simulink model "nms_3Dmodel"  (R2017b)
settings: Solver=ode15s  StartTime=0.0  StopTime=t_end  FixedStep=1e-3  RelTol=1e-3  AbsTol=1e-4  EnableMultiTasking=on
InitFcn:
  | runScripts;
values from neighbouring files (symbols this model uses):
  ankle_height = 0.08    [nms_MechInit.m]
  ankleIMP = param(91+length(paramIC_opt):93+length(paramIC_opt))    [runScripts.m]
  c = 0.05    [IID_nms_MechInit.m]    (also in nms_MechInit.m)
  c_jointstop = 0.3 / (pi/180)    (= 17.1887338539)    [IID_nms_MechInit.m]    (also in nms_MechInit.m)
  CtrlPar_FP = [alpha0 alpha_cd alpha_cv]    [setCtrlPar.m]
  CtrlPar_FP_R = [R_hipR0 R_hipR_cd R_hipR_cv]    [setCtrlPar.m]
  CtrlPar_LL = l_clr    [setCtrlPar.m]
  CtrlPar_St = [StPreStim St_M1 St_M2 St_M3 St_M4 St_M5 St_M11]    [setCtrlPar.m]
  CtrlPar_St_R = [R_StPreStim R_St_M1 R_St_M3 R_St_M4]    [setCtrlPar.m]
  CtrlPar_Sw = [SwPreStim SwPhasePari SwPhaseParii SwCtrlPar_H SwCtrlPar_A      SwCtrlPar_Ki SwCtrlPar_Kii SwCtrlPar_Kiii SwCtrlPar_StP]    [setCtrlPar.m]
  CtrlPar_Sw_R = [R_SwPreStim R_Sw_M6]    [setCtrlPar.m]
  CtrlPar_theta0 = parBlCtrl(1)      *1*pi/180    [setCtrlPar.m]
  CtrlPar_Tr = [Tr_St_sup Tr_Sw]    [setCtrlPar.m]
  CtrlPar_Tr_R = [R_Tr_St_sup R_Tr_Sw]    [setCtrlPar.m]
  D12_F = 0.16    [IID_nms_MechInit.m]    (also in nms_MechInit.m)
  D12_S = L_S    (= 0.5)    [IID_nms_MechInit.m]    (also in nms_MechInit.m = 0.46)
  D12_T = L_T    (= 0.5)    [IID_nms_MechInit.m]    (also in nms_MechInit.m = 0.46)
  D12z_T = 0.1* scalorFactor    (= 0.1)    [nms_MechInit.m]
  D13_F = 0.20    (= 0.2)    [IID_nms_MechInit.m]    (also in nms_MechInit.m)
  D1G_F = 0.14    [IID_nms_MechInit.m]    (also in nms_MechInit.m)
  D1G_HAT = 0.35    [IID_nms_MechInit.m]    (also in nms_MechInit.m)
  D1G_S = 0.3    [IID_nms_MechInit.m]    (also in nms_MechInit.m = 0.28)
  D1G_T = 0.3    [IID_nms_MechInit.m]    (also in nms_MechInit.m = 0.28)
  D1Gy_F = ankle_height*D1G_F/D12_F    (= 0.07)    [nms_MechInit.m]
  d_fBall = 0.1    [nms_MechInit.m]
  d_fHeel = 0.05    [nms_MechInit.m]
  DeltaThRef = 5e-3    (= 0.005)    [IID_nms_MechInit.m]    (also in nms_MechInit.m)
  Dist_LM23_PH = 0    [setDistPar.m]
  Dist_LM34_PH = 0    [setDistPar.m]
  Dist_On = 1    [IID_setDistPar.m]    (also in setDistPar.m)
  Dist_PDur = 0.15    [IID_setDistPar.m]    (also in setDistPar.m)
  Dist_RM23_PH = 0    [setDistPar.m]
  Dist_RM34_PH = 0    [setDistPar.m]
  Dist_StartTime = 15    [IID_setDistPar.m]    (also in setDistPar.m)
  Dist_xyzHAT_front_PH = 0    [setDistPar.m]
  Dist_xyzHAT_sag_PH = 0    [IID_setDistPar.m]    (also in setDistPar.m)
  Dist_xyzLAnkle_PH = 0    [setDistPar.m]
  Dist_xyzRAnkle_PH = 0    [setDistPar.m]
  eref = 0.04    [IID_nms_MechInit.m]    (also in nms_MechInit.m)
  FmaxBFSH = 350    [nms_MechInit.m]
  FmaxGAS = 1500    [IID_nms_MechInit.m]    (also in nms_MechInit.m)
  FmaxGLU = 1500    [IID_nms_MechInit.m]    (also in nms_MechInit.m)
  FmaxHAB = 3000    [nms_MechInit.m]
  FmaxHAD = 4500    [nms_MechInit.m]
  FmaxHAM = 3000    [IID_nms_MechInit.m]    (also in nms_MechInit.m)
  FmaxHFL = 2000    [IID_nms_MechInit.m]    (also in nms_MechInit.m)
  FmaxRF = 1200    [nms_MechInit.m]
  FmaxSOL = 4000    [IID_nms_MechInit.m]    (also in nms_MechInit.m)
  FmaxTA = 800    [IID_nms_MechInit.m]    (also in nms_MechInit.m)
  FmaxVAS = 6000    [IID_nms_MechInit.m]    (also in nms_MechInit.m)
  In_F = 0.005    [IID_nms_MechInit.m]    (also in nms_MechInit.m)
  In_HAT = 3    [IID_nms_MechInit.m]    (also in nms_MechInit.m = 2.5)
  In_S = 0.05    [IID_nms_MechInit.m]    (also in nms_MechInit.m)
  In_T = 0.15    [IID_nms_MechInit.m]    (also in nms_MechInit.m)
  init_a_tgt = 70*pi/180    (= 1.2217304764)    [setInitPar.m]
  init_a_tgtR = 90*pi/180    (= 1.57079632679)    [setInitPar.m]
  Inx_F = 0.0007    [nms_MechInit.m]
  Inx_HAT = 1.0    (= 1)    [nms_MechInit.m]
  Inx_S = 0.003    [nms_MechInit.m]
  Inx_T = 0.03    [nms_MechInit.m]
  Iny_F = 0.005    [nms_MechInit.m]
  Iny_HAT = 4.0    (= 4)    [nms_MechInit.m]
  Iny_S = 0.05    [nms_MechInit.m]
  Iny_T = 0.15    [nms_MechInit.m]
  K = 5    [IID_nms_MechInit.m]    (also in nms_MechInit.m)
  k_gn = k_gn/2    (= 39240)    [nms_MechInit.m]
  k_gt = k_gt/2    (= 3924)    [nms_MechInit.m]
  k_pressure = m_HAT * 9.81 / DeltaThRef    (= 104967)    [IID_nms_MechInit.m]    (also in nms_MechInit.m)
  leg_l = [D12_T D12_S]    [nms_MechInit.m]
  LongDelay = 0.020    (= 0.02)    [IID_setCtrlPar.m]    (also in nms_MechInit.m = 0.01)
  LongLoopDelay = 0.030    (= 0.03)    [nms_MechInit.m]
  loptBFSH = 0.12    [nms_MechInit.m]
  loptGAS = 0.05    [IID_nms_MechInit.m]    (also in nms_MechInit.m)
  loptGLU = 0.11    [IID_nms_MechInit.m]    (also in nms_MechInit.m)
  loptHAB = 0.09    [nms_MechInit.m]
  loptHAD = 0.10    (= 0.1)    [nms_MechInit.m]
  loptHAM = 0.10    (= 0.1)    [IID_nms_MechInit.m]    (also in nms_MechInit.m)
  loptHFL = 0.11    [IID_nms_MechInit.m]    (also in nms_MechInit.m)
  loptRF = 0.08    [nms_MechInit.m]
  loptSOL = 0.04    [IID_nms_MechInit.m]    (also in nms_MechInit.m)
  loptTA = 0.06    [IID_nms_MechInit.m]    (also in nms_MechInit.m)
  loptVAS = 0.08    [IID_nms_MechInit.m]    (also in nms_MechInit.m)
  lslackBFSH = 0.10    (= 0.1)    [nms_MechInit.m]
  lslackGAS = 0.40    (= 0.4)    [IID_nms_MechInit.m]    (also in nms_MechInit.m)
  lslackGLU = 0.13    [IID_nms_MechInit.m]    (also in nms_MechInit.m)
  lslackHAB = 0.07    [nms_MechInit.m]
  lslackHAD = 0.18    [nms_MechInit.m]
  lslackHAM = 0.31    [IID_nms_MechInit.m]    (also in nms_MechInit.m)
  lslackHFL = 0.10    (= 0.1)    [IID_nms_MechInit.m]    (also in nms_MechInit.m)
  lslackRF = 0.35    [nms_MechInit.m]
  lslackSOL = 0.26    [IID_nms_MechInit.m]    (also in nms_MechInit.m)
  lslackTA = 0.24    [IID_nms_MechInit.m]    (also in nms_MechInit.m)
  lslackVAS = 0.23    [IID_nms_MechInit.m]    (also in nms_MechInit.m)
  m_F = 1.25    [IID_nms_MechInit.m]    (also in nms_MechInit.m)
  m_HAT = 53.5    [IID_nms_MechInit.m]    (also in nms_MechInit.m)
  m_S = 3.5    [IID_nms_MechInit.m]    (also in nms_MechInit.m)
  m_T = 8.5    [IID_nms_MechInit.m]    (also in nms_MechInit.m)
  m_Total = m_F*2+m_S*2+m_T*2+m_HAT    (= 80)    [IID_nms_MechInit.m]    (also in nms_MechInit.m)
  massBFSH = 2    [nms_MechInit.m]
  massGAS = 0.45    [IID_nms_MechInit.m]    (also in nms_MechInit.m)
  massGLU = 1.4    [IID_nms_MechInit.m]    (also in nms_MechInit.m)
  massHAB = 1.145    [nms_MechInit.m]
  massHAD = 1.91    [nms_MechInit.m]
  massHAM = 1.82    [IID_nms_MechInit.m]    (also in nms_MechInit.m)
  massHFL = 1.87    [IID_nms_MechInit.m]    (also in nms_MechInit.m)
  massRF = 1    [nms_MechInit.m]
  massSOL = 1.36    [IID_nms_MechInit.m]    (also in nms_MechInit.m)
  massTA = 0.29    [IID_nms_MechInit.m]    (also in nms_MechInit.m)
  massVAS = 2.91    [IID_nms_MechInit.m]    (also in nms_MechInit.m)
  MidDelay = 0.010    (= 0.01)    [IID_setCtrlPar.m]    (also in nms_MechInit.m = 0.005)
  mu_slide = 0.8    [IID_nms_MechInit.m]    (also in nms_MechInit.m)
  mu_stick = 0.9    [IID_nms_MechInit.m]    (also in nms_MechInit.m)
  N = 1.5    [IID_nms_MechInit.m]    (also in cmaes_parfor.m = size(x,1); nms_MechInit.m)
  Passive_ankle = 1    [runScripts.m]
  phi12_LowLimit = 70*pi/180    (= 1.2217304764)    [IID_nms_MechInit.m]    (also in nms_MechInit.m)
  phi12_UpLimit = 130*pi/180    (= 2.26892802759)    [IID_nms_MechInit.m]    (also in nms_MechInit.m)
  phi23_UpLimit = 175*pi/180    (= 3.05432619099)    [IID_nms_MechInit.m]    (also in nms_MechInit.m)
  phi34_UpLimit = 230*pi/180    (= 4.01425727959)    [IID_nms_MechInit.m]    (also in nms_MechInit.m)
  phi34R_LowLimit = -15*pi/180    (= -0.261799387799)    [nms_MechInit.m]
  phi34R_UpLimit = 50*pi/180    (= 0.872664625997)    [nms_MechInit.m]
  ... (+114 more)
undefined symbols (not defined in the file or in its folder): magnitude, sgn
libraries: mblibv1 x104, simulink x50, simulink_extras x38, nmc x30
(part 5 of 16)

== system nms_3Dmodel/Body Mechanics Layer/LLHeelCnt5 ==
  note: 3D Ground Interaction Model
  PosContra : Inport
  3D Contact : Subsystem
  Body Actuator : mblibv1/Sensors &  Actuators/Body Actuator  UpdateFromCAD=off  PhysicalDomain=Mechanical  PortType=blob  ActuationStyle=Force  AngleUnits=deg  ArcVelocityUnits=deg/s  ArcAccelerationUnits=deg/s^2  CoordPositionUnits=m  VelocityUnits=m/s  AccelerationUnits=m/s^2  ForceUnits=N  TorqueUnits=N*m  ActiveIO=on  Width=3  DialogClass=MechanicalActuatorBlock  ReferenceFrame=Absolute (World)  Angle=off  CoordPosition=on  Force=on  Torque=off
      settings: SourceProductName=Simscape Multibody  SourceProductBaseCode=MS
  Body Sensor : mblibv1/Sensors &  Actuators/Body Sensor  UpdateFromCAD=off  PhysicalDomain=Mechanical  PortType=blob  Muxed=off  Pose=off  Angle=on  AngleUnits=deg  ArcVelocity=off  ArcVelocityUnits=deg/s  ArcAcceleration=off  ArcAccelerationUnits=deg/s^2  CoordPosition=on  CoordPositionUnits=m  Velocity=on  VelocityUnits=m/s  Acceleration=off  AccelerationUnits=m/s^2  Quaternion=on  QuaternionDT=off  QuaternionDDT=off  QuaternionUnits=off  OutputVector=[ 3 3 ]  ActiveIO=on  Width=6  DialogClass=MechanicalSensorBlock  ReferenceFrame=Absolute (World)
      settings: SourceProductName=Simscape Multibody  SourceProductBaseCode=MS
  Demux1 : Demux  Outputs=3
  GroundFunction : nmc/GroundFunction
      settings: SourceProductName=Neuro Muscular Controller Library
  Mechanical Branching Bar : mblibv1/Utilities/Mechanical Branching Bar  LConnTagsString=_newl0  RConnTagsString=SA0|SA1  UpdateFromCAD=off  DialogClass=MechanicalBranchingBarBlock  NumSAPorts=2
      settings: SourceProductName=Simscape Multibody  SourceProductBaseCode=MS
  Mux : Mux  Inputs=3
  Sum : Sum  Inputs=|+-
  Sum1 : Sum
  Terminator : Terminator
  contact? : simulink/Logic and Bit Operations/Compare To Zero  relop=<=  OutDataTypeStr=boolean
  y : Selector  InputPortWidth=3  IndexOptions=Index vector (dialog)  Indices=2  OutputSizes=1
  F : PMIOPort  Port=1  Side=Left
  RBallCnt : Outport
  tag scope: GRF_LLHeelCnt5=global
  wires:
  GroundFunction/2 -> 3D Contact/2(nVec [m m m])
  GroundFunction/1 -> Mux/2, Sum/2
  Demux1/2 -> Terminator/1
  Demux1/3 -> Mux/3
  Demux1/1 -> Mux/1
  Mux/1 -> 3D Contact/1(RefPt [m m m])  "Reference Point RefPt"
  y/1 -> Sum/1
  Sum/1 -> contact?/1
  3D Contact/2(FtVec [N N N]) -> Sum1/2
  3D Contact/1(FnVec [N N N]) -> Sum1/1
  Body Sensor/2 -> 3D Contact/4(vVec [m/s m/s m/s])
  Body Sensor/1 -> y/1, Demux1/1, 3D Contact/3(pVec [m m m])  "pos"
  contact?/1 -> RBallCnt/1, 3D Contact/Enable  "cnt"
  PosContra/1 -> GroundFunction/1
  Sum1/1 -> [GRF_LLHeelCnt5], Body Actuator/1
  connections:
  Mechanical Branching Bar/RConn1 -- Body Sensor/LConn1
  Mechanical Branching Bar/RConn2 -- Body Actuator/RConn1
  F/RConn1 -- Mechanical Branching Bar/LConn1

== system nms_3Dmodel/Body Mechanics Layer/LLHeelCnt6 ==
  note: 3D Ground Interaction Model
  PosContra : Inport
  3D Contact : Subsystem
  Body Actuator : mblibv1/Sensors &  Actuators/Body Actuator  UpdateFromCAD=off  PhysicalDomain=Mechanical  PortType=blob  ActuationStyle=Force  AngleUnits=deg  ArcVelocityUnits=deg/s  ArcAccelerationUnits=deg/s^2  CoordPositionUnits=m  VelocityUnits=m/s  AccelerationUnits=m/s^2  ForceUnits=N  TorqueUnits=N*m  ActiveIO=on  Width=3  DialogClass=MechanicalActuatorBlock  ReferenceFrame=Absolute (World)  Angle=off  CoordPosition=on  Force=on  Torque=off
      settings: SourceProductName=Simscape Multibody  SourceProductBaseCode=MS
  Body Sensor : mblibv1/Sensors &  Actuators/Body Sensor  UpdateFromCAD=off  PhysicalDomain=Mechanical  PortType=blob  Muxed=off  Pose=off  Angle=on  AngleUnits=deg  ArcVelocity=off  ArcVelocityUnits=deg/s  ArcAcceleration=off  ArcAccelerationUnits=deg/s^2  CoordPosition=on  CoordPositionUnits=m  Velocity=on  VelocityUnits=m/s  Acceleration=off  AccelerationUnits=m/s^2  Quaternion=on  QuaternionDT=off  QuaternionDDT=off  QuaternionUnits=off  OutputVector=[ 3 3 ]  ActiveIO=on  Width=6  DialogClass=MechanicalSensorBlock  ReferenceFrame=Absolute (World)
      settings: SourceProductName=Simscape Multibody  SourceProductBaseCode=MS
  Demux1 : Demux  Outputs=3
  GroundFunction : nmc/GroundFunction
      settings: SourceProductName=Neuro Muscular Controller Library
  Mechanical Branching Bar : mblibv1/Utilities/Mechanical Branching Bar  LConnTagsString=_newl0  RConnTagsString=SA0|SA1  UpdateFromCAD=off  DialogClass=MechanicalBranchingBarBlock  NumSAPorts=2
      settings: SourceProductName=Simscape Multibody  SourceProductBaseCode=MS
  Mux : Mux  Inputs=3
  Sum : Sum  Inputs=|+-
  Sum1 : Sum
  Terminator : Terminator
  contact? : simulink/Logic and Bit Operations/Compare To Zero  relop=<=  OutDataTypeStr=boolean
  y : Selector  InputPortWidth=3  IndexOptions=Index vector (dialog)  Indices=2  OutputSizes=1
  F : PMIOPort  Port=1  Side=Left
  RBallCnt : Outport
  tag scope: GRF_LLHeelCnt6=global
  wires:
  GroundFunction/2 -> 3D Contact/2(nVec [m m m])
  GroundFunction/1 -> Mux/2, Sum/2
  Demux1/2 -> Terminator/1
  Demux1/3 -> Mux/3
  Demux1/1 -> Mux/1
  Mux/1 -> 3D Contact/1(RefPt [m m m])  "Reference Point RefPt"
  y/1 -> Sum/1
  Sum/1 -> contact?/1
  3D Contact/2(FtVec [N N N]) -> Sum1/2
  3D Contact/1(FnVec [N N N]) -> Sum1/1
  Body Sensor/2 -> 3D Contact/4(vVec [m/s m/s m/s])
  Body Sensor/1 -> y/1, Demux1/1, 3D Contact/3(pVec [m m m])  "pos"
  contact?/1 -> RBallCnt/1, 3D Contact/Enable  "cnt"
  PosContra/1 -> GroundFunction/1
  Sum1/1 -> [GRF_LLHeelCnt6], Body Actuator/1
  connections:
  Mechanical Branching Bar/RConn1 -- Body Sensor/LConn1
  Mechanical Branching Bar/RConn2 -- Body Actuator/RConn1
  F/RConn1 -- Mechanical Branching Bar/LConn1

== system nms_3Dmodel/Body Mechanics Layer/LLHeelCnt7 ==
  note: 3D Ground Interaction Model
  3D Contact : Subsystem
  Body Actuator : mblibv1/Sensors &  Actuators/Body Actuator  UpdateFromCAD=off  PhysicalDomain=Mechanical  PortType=blob  ActuationStyle=Force  AngleUnits=deg  ArcVelocityUnits=deg/s  ArcAccelerationUnits=deg/s^2  CoordPositionUnits=m  VelocityUnits=m/s  AccelerationUnits=m/s^2  ForceUnits=N  TorqueUnits=N*m  ActiveIO=on  Width=3  DialogClass=MechanicalActuatorBlock  ReferenceFrame=Absolute (World)  Angle=off  CoordPosition=on  Force=on  Torque=off
      settings: SourceProductName=Simscape Multibody  SourceProductBaseCode=MS
  Body Sensor : mblibv1/Sensors &  Actuators/Body Sensor  UpdateFromCAD=off  PhysicalDomain=Mechanical  PortType=blob  Muxed=off  Pose=off  Angle=on  AngleUnits=deg  ArcVelocity=off  ArcVelocityUnits=deg/s  ArcAcceleration=off  ArcAccelerationUnits=deg/s^2  CoordPosition=on  CoordPositionUnits=m  Velocity=on  VelocityUnits=m/s  Acceleration=off  AccelerationUnits=m/s^2  Quaternion=on  QuaternionDT=off  QuaternionDDT=off  QuaternionUnits=off  OutputVector=[ 3 3 ]  ActiveIO=on  Width=6  DialogClass=MechanicalSensorBlock  ReferenceFrame=Absolute (World)
      settings: SourceProductName=Simscape Multibody  SourceProductBaseCode=MS
  Demux1 : Demux  Outputs=3
  GroundFunction : nmc/GroundFunction
      settings: SourceProductName=Neuro Muscular Controller Library
  Mechanical Branching Bar : mblibv1/Utilities/Mechanical Branching Bar  LConnTagsString=_newl0  RConnTagsString=SA0|SA1  UpdateFromCAD=off  DialogClass=MechanicalBranchingBarBlock  NumSAPorts=2
      settings: SourceProductName=Simscape Multibody  SourceProductBaseCode=MS
  Mux : Mux  Inputs=3
  Sum : Sum  Inputs=|+-
  Sum1 : Sum
  Terminator : Terminator
  contact? : simulink/Logic and Bit Operations/Compare To Zero  relop=<=  OutDataTypeStr=boolean
  y : Selector  InputPortWidth=3  IndexOptions=Index vector (dialog)  Indices=2  OutputSizes=1
  F : PMIOPort  Port=1  Side=Left
  RBallCnt : Outport
  RBallCnt1 : Outport  Port=2
  tag scope: GRF_LLHeelCnt7=global
  wires:
  contact?/1 -> 3D Contact/Enable, RBallCnt/1  "cnt"
  Body Sensor/1 -> RBallCnt1/1, GroundFunction/1, 3D Contact/3(pVec [m m m]), Demux1/1, y/1  "pos"
  Body Sensor/2 -> 3D Contact/4(vVec [m/s m/s m/s])
  3D Contact/1(FnVec [N N N]) -> Sum1/1
  3D Contact/2(FtVec [N N N]) -> Sum1/2
  Sum/1 -> contact?/1
  y/1 -> Sum/1
  Mux/1 -> 3D Contact/1(RefPt [m m m])  "Reference Point RefPt"
  Demux1/1 -> Mux/1
  Demux1/3 -> Mux/3
  Demux1/2 -> Terminator/1
  GroundFunction/1 -> Sum/2, Mux/2
  GroundFunction/2 -> 3D Contact/2(nVec [m m m])
  Sum1/1 -> [GRF_LLHeelCnt7], Body Actuator/1
  connections:
  F/RConn1 -- Mechanical Branching Bar/LConn1
  Mechanical Branching Bar/RConn2 -- Body Actuator/RConn1
  Mechanical Branching Bar/RConn1 -- Body Sensor/LConn1

== system nms_3Dmodel/Body Mechanics Layer/LLHeelCnt8 ==
  note: 3D Ground Interaction Model
  3D Contact : Subsystem
  Body Actuator : mblibv1/Sensors &  Actuators/Body Actuator  UpdateFromCAD=off  PhysicalDomain=Mechanical  PortType=blob  ActuationStyle=Force  AngleUnits=deg  ArcVelocityUnits=deg/s  ArcAccelerationUnits=deg/s^2  CoordPositionUnits=m  VelocityUnits=m/s  AccelerationUnits=m/s^2  ForceUnits=N  TorqueUnits=N*m  ActiveIO=on  Width=3  DialogClass=MechanicalActuatorBlock  ReferenceFrame=Absolute (World)  Angle=off  CoordPosition=on  Force=on  Torque=off
      settings: SourceProductName=Simscape Multibody  SourceProductBaseCode=MS
  Body Sensor : mblibv1/Sensors &  Actuators/Body Sensor  UpdateFromCAD=off  PhysicalDomain=Mechanical  PortType=blob  Muxed=off  Pose=off  Angle=on  AngleUnits=deg  ArcVelocity=off  ArcVelocityUnits=deg/s  ArcAcceleration=off  ArcAccelerationUnits=deg/s^2  CoordPosition=on  CoordPositionUnits=m  Velocity=on  VelocityUnits=m/s  Acceleration=off  AccelerationUnits=m/s^2  Quaternion=on  QuaternionDT=off  QuaternionDDT=off  QuaternionUnits=off  OutputVector=[ 3 3 ]  ActiveIO=on  Width=6  DialogClass=MechanicalSensorBlock  ReferenceFrame=Absolute (World)
      settings: SourceProductName=Simscape Multibody  SourceProductBaseCode=MS
  Demux1 : Demux  Outputs=3
  GroundFunction : nmc/GroundFunction
      settings: SourceProductName=Neuro Muscular Controller Library
  Mechanical Branching Bar : mblibv1/Utilities/Mechanical Branching Bar  LConnTagsString=_newl0  RConnTagsString=SA0|SA1  UpdateFromCAD=off  DialogClass=MechanicalBranchingBarBlock  NumSAPorts=2
      settings: SourceProductName=Simscape Multibody  SourceProductBaseCode=MS
  Mux : Mux  Inputs=3
  Sum : Sum  Inputs=|+-
  Sum1 : Sum
  Terminator : Terminator
  contact? : simulink/Logic and Bit Operations/Compare To Zero  relop=<=  OutDataTypeStr=boolean
  y : Selector  InputPortWidth=3  IndexOptions=Index vector (dialog)  Indices=2  OutputSizes=1
  F : PMIOPort  Port=1  Side=Left
  RBallCnt : Outport
  RBallCnt1 : Outport  Port=2
  tag scope: GRF_LLHeelCnt8=global
  wires:
  contact?/1 -> 3D Contact/Enable, RBallCnt/1  "cnt"
  Body Sensor/1 -> RBallCnt1/1, GroundFunction/1, 3D Contact/3(pVec [m m m]), Demux1/1, y/1  "pos"
  Body Sensor/2 -> 3D Contact/4(vVec [m/s m/s m/s])
  3D Contact/1(FnVec [N N N]) -> Sum1/1
  3D Contact/2(FtVec [N N N]) -> Sum1/2
  Sum/1 -> contact?/1
  y/1 -> Sum/1
  Mux/1 -> 3D Contact/1(RefPt [m m m])  "Reference Point RefPt"
  Demux1/1 -> Mux/1
  Demux1/3 -> Mux/3
  Demux1/2 -> Terminator/1
  GroundFunction/1 -> Sum/2, Mux/2
  GroundFunction/2 -> 3D Contact/2(nVec [m m m])
  Sum1/1 -> [GRF_LLHeelCnt8], Body Actuator/1
  connections:
  F/RConn1 -- Mechanical Branching Bar/LConn1
  Mechanical Branching Bar/RConn2 -- Body Actuator/RConn1
  Mechanical Branching Bar/RConn1 -- Body Sensor/LConn1

== system nms_3Dmodel/Body Mechanics Layer/Left Leg Load ==
  dxThigh [m] : Inport
  FB Gain1 : Gain  Gain=1/DeltaThRef  SaturateOnIntegerOverflow=on  OutDataTypeStr=Inherit: Same as input  ParamDataTypeStr=Inherit: Same as input
  Saturation11 : Saturate  UpperLimit=inf  LowerLimit=0  ZeroCross=off
  smooth2 : TransferFcn  Denominator=[0.02 1]
  LLoad [F] : Outport
  wires:
  Saturation11/1 -> FB Gain1/1
  smooth2/1 -> Saturation11/1
  FB Gain1/1 -> LLoad [F]/1
  dxThigh [m]/1 -> smooth2/1

== system nms_3Dmodel/Body Mechanics Layer/Left Thigh Sensor Sheet ==
  note: Inner Segment Pressure Sheet
  Gain3 : Gain  Gain=k_pressure
  Gain4 : Gain  Gain=1/v_max_pressure
  Inner Thigh Shift Joint : mblibv1/Joints/Prismatic  LConnTagsString=__newl0|SA1|SA2  RConnTagsString=__newr0|SA1  UpdateFromCAD=off  NumSAPorts=3  CutJoint=off  MarkAsCut=off  Primitives=prismatic  PrimitiveProps=P1$WORLD$[1 0 0]$prismatic  DialogClass=JointBlock  P1Axis=[1 0 0]
      settings: SourceProductName=Simscape Multibody  SourceProductBaseCode=MS
  Left Thigh Sensor Sheet IC : mblibv1/Sensors &  Actuators/Joint Initial Condition  UpdateFromCAD=off  LeftPortType=blob  RightPortType=blob  PhysicalDomain=mechanical  DialogClass=InitialConditionBlock  InitialConditions=P1$true$0$m$rad$0$m/s$rad/s#P2$false$0$m$rad$0$m/s$rad/s#P3$false$0$m$rad$0$m/s$rad/s#R1$false$0$m$rad$0$m/s$rad/s#R2$false$0$m$rad$0$m/s$rad/s#R3$false$0$m$rad$0$m/s$rad/s#S$false$0$m$rad$0$m/s$rad/s  P1PIC=0  P1VIC=0  P2PIC=0  P2VIC=0  P3PIC=0  P3VIC=0  R1PIC=0  R1VIC=0  R2PIC=0  R2VIC=0  R3PIC=0  R3VIC=0  SPIC=0  SVIC=0
      settings: SourceProductName=Simscape Multibody  SourceProductBaseCode=MS
  Mux1 : Mux  Inputs=2
  Pressure Sheet Reaction Force : Fcn  Expr=-u(1) * (1+sgn(u(1))*u(2))
  Thigh Actuator : mblibv1/Sensors &  Actuators/Joint Actuator  UpdateFromCAD=off  PhysicalDomain=Mechanical  PortType=blob  ActuationStyle=Force  AngleUnits=deg  ArcVelocityUnits=deg/s  ArcAccelerationUnits=deg/s^2  CoordPositionUnits=m  VelocityUnits=m/s  AccelerationUnits=m/s^2  ForceUnits=N  TorqueUnits=N-m  ActiveIO=on  Width=1  DialogClass=MechanicalActuatorBlock  Primitive=P1  ReferenceFrame=Absolute (INERTIAL)
      settings: SourceProductName=Simscape Multibody  SourceProductBaseCode=MS
  Thigh Sensor : mblibv1/Sensors &  Actuators/Joint Sensor  UpdateFromCAD=off  PhysicalDomain=Mechanical  PortType=blob  Muxed=off  Pose=off  Angle=on  AngleUnits=deg  ArcVelocity=off  ArcVelocityUnits=deg/s  ArcAcceleration=off  ArcAccelerationUnits=deg/s^2  CoordPosition=on  CoordPositionUnits=m  Velocity=on  VelocityUnits=m/s  Acceleration=off  AccelerationUnits=m/s^2  Quaternion=on  QuaternionDT=off  QuaternionDDT=off  QuaternionUnits=off  OutputVector=[ 1 1 ]  ActiveIO=on  Width=2  DialogClass=MechanicalSensorBlock  Primitive=P1  Force=off  ForceUnits=N  Torque=off  TorqueUnits=N-m  ReferenceFrame=Absolute (INERTIAL)  ReactionSensedSide=Base  ReactionReferenceFrame=Absolute (World)  ReactionForce=off  ReactionForceUnits=N  ReactionMoment=off  ReactionMomentUnits=N-m
      settings: SourceProductName=Simscape Multibody  SourceProductBaseCode=MS
  B : PMIOPort  Tag=PMCPort  Port=1  Side=Left
  F : PMIOPort  Tag=PMCPort  Port=2  Side=Right
  dx : Outport
  wires:
  Thigh Sensor/1 -> Gain3/1, dx/1
  Thigh Sensor/2 -> Gain4/1
  Mux1/1 -> Pressure Sheet Reaction Force/1
  Gain3/1 -> Mux1/1
  Gain4/1 -> Mux1/2
  Pressure Sheet Reaction Force/1 -> Thigh Actuator/1
  connections:
  B/RConn1 -- Inner Thigh Shift Joint/LConn1
  F/RConn1 -- Inner Thigh Shift Joint/RConn1
  Thigh Sensor/LConn1 -- Inner Thigh Shift Joint/LConn2
  Inner Thigh Shift Joint/RConn2 -- Thigh Actuator/RConn1
  Left Thigh Sensor Sheet IC/RConn1 -- Inner Thigh Shift Joint/LConn3

== system nms_3Dmodel/Body Mechanics Layer/RAnkle ==
  note: 3D Ground Interaction Model
  Dist : Inport
  Body Actuator : mblibv1/Sensors &  Actuators/Body Actuator  UpdateFromCAD=off  PhysicalDomain=Mechanical  PortType=blob  ActuationStyle=Force  AngleUnits=deg  ArcVelocityUnits=deg/s  ArcAccelerationUnits=deg/s^2  CoordPositionUnits=m  VelocityUnits=m/s  AccelerationUnits=m/s^2  ForceUnits=N  TorqueUnits=N*m  ActiveIO=on  Width=3  DialogClass=MechanicalActuatorBlock  ReferenceFrame=Local (Body CS)  Angle=off  CoordPosition=on  Force=on  Torque=off
      settings: SourceProductName=Simscape Multibody  SourceProductBaseCode=MS
  Constant : Constant  Value=0
  Gain : Gain  Gain=-1
  Mechanical Branching Bar : mblibv1/Utilities/Mechanical Branching Bar  LConnTagsString=_newl0  RConnTagsString=SA0|SA1  UpdateFromCAD=off  DialogClass=MechanicalBranchingBarBlock  NumSAPorts=2
      settings: SourceProductName=Simscape Multibody  SourceProductBaseCode=MS
  Mux : Mux  Inputs=3
  Right Heel Sensor15 : mblibv1/Sensors &  Actuators/Body Sensor  UpdateFromCAD=off  PhysicalDomain=Mechanical  PortType=blob  Muxed=off  Pose=off  Angle=on  AngleUnits=deg  ArcVelocity=off  ArcVelocityUnits=deg/s  ArcAcceleration=off  ArcAccelerationUnits=deg/s^2  CoordPosition=on  CoordPositionUnits=m  Velocity=off  VelocityUnits=m/s  Acceleration=off  AccelerationUnits=m/s^2  Quaternion=on  QuaternionDT=off  QuaternionDDT=off  QuaternionUnits=off  OutputVector=[ 3 3 ]  ActiveIO=on  Width=3  DialogClass=MechanicalSensorBlock  ReferenceFrame=Absolute (World)
      settings: SourceProductName=Simscape Multibody  SourceProductBaseCode=MS
  F : PMIOPort  Port=1  Side=Left
  Pos : Outport
  wires:
  Right Heel Sensor15/1 -> Pos/1  "pos"
  Mux/1 -> Body Actuator/1
  Dist/1 -> Gain/1
  Gain/1 -> Mux/2
  Constant/1 -> Mux/3, Mux/1
  connections:
  F/RConn1 -- Mechanical Branching Bar/LConn1
  Mechanical Branching Bar/RConn2 -- Body Actuator/RConn1
  Right Heel Sensor15/LConn1 -- Mechanical Branching Bar/RConn1

== system nms_3Dmodel/Body Mechanics Layer/RLBall Cnt1 ==
  note: 3D Ground Interaction Model
  Dist_sag : Inport
  Dist_front : Inport  Port=2
  Body Actuator : mblibv1/Sensors &  Actuators/Body Actuator  UpdateFromCAD=off  PhysicalDomain=Mechanical  PortType=blob  ActuationStyle=Force  AngleUnits=deg  ArcVelocityUnits=deg/s  ArcAccelerationUnits=deg/s^2  CoordPositionUnits=m  VelocityUnits=m/s  AccelerationUnits=m/s^2  ForceUnits=N  TorqueUnits=N*m  ActiveIO=on  Width=3  DialogClass=MechanicalActuatorBlock  ReferenceFrame=Local (Body CS)  Angle=off  CoordPosition=on  Force=on  Torque=off
      settings: SourceProductName=Simscape Multibody  SourceProductBaseCode=MS
  Gain : Gain  Gain=-1
  Mechanical Branching Bar : mblibv1/Utilities/Mechanical Branching Bar  LConnTagsString=_newl0  RConnTagsString=SA0|SA1  UpdateFromCAD=off  DialogClass=MechanicalBranchingBarBlock  NumSAPorts=2
      settings: SourceProductName=Simscape Multibody  SourceProductBaseCode=MS
  Mux : Mux  Inputs=3
  Product : Product
  Product1 : Product
  Right Heel Sensor5 : mblibv1/Sensors &  Actuators/Body Sensor  UpdateFromCAD=off  PhysicalDomain=Mechanical  PortType=blob  Muxed=off  Pose=on  Angle=on  AngleUnits=deg  ArcVelocity=off  ArcVelocityUnits=deg/s  ArcAcceleration=off  ArcAccelerationUnits=deg/s^2  CoordPosition=on  CoordPositionUnits=m  Velocity=off  VelocityUnits=m/s  Acceleration=off  AccelerationUnits=m/s^2  Quaternion=on  QuaternionDT=off  QuaternionDDT=off  QuaternionUnits=off  OutputVector=[ 3 3 ]  ActiveIO=on  Width=12  DialogClass=MechanicalSensorBlock  ReferenceFrame=Absolute (World)
      settings: SourceProductName=Simscape Multibody  SourceProductBaseCode=MS
  Trigonometric Function : Trigonometry  Operator=cos
  Trigonometric Function1 : Trigonometry
  F : PMIOPort  Port=1  Side=Left
  Pos : Outport
  Rot : Outport  Port=2
  wires:
  Right Heel Sensor5/1 -> Pos/1  "pos"
  Mux/1 -> Body Actuator/1
  Dist_front/1 -> Mux/3
  Right Heel Sensor5/2 -> Rot/1
  [theta] -> Trigonometric Function/1, Trigonometric Function1/1
  Dist_sag/1 -> Product1/2, Product/2
  Trigonometric Function/1 -> Product/1
  Product/1 -> Gain/1
  Gain/1 -> Mux/2
  Trigonometric Function1/1 -> Product1/1
  Product1/1 -> Mux/1
  connections:
  F/RConn1 -- Mechanical Branching Bar/LConn1
  Mechanical Branching Bar/RConn2 -- Body Actuator/RConn1
  Mechanical Branching Bar/RConn1 -- Right Heel Sensor5/LConn1

== system nms_3Dmodel/Body Mechanics Layer/Right Leg Load ==
  dxThigh [m] : Inport
  FB Gain1 : Gain  Gain=1/DeltaThRef  SaturateOnIntegerOverflow=on  OutDataTypeStr=Inherit: Same as input  ParamDataTypeStr=Inherit: Same as input
  Saturation11 : Saturate  UpperLimit=inf  LowerLimit=0  ZeroCross=off
  smooth2 : TransferFcn  Denominator=[0.02 1]
  LLoad [F] : Outport
  wires:
  Saturation11/1 -> FB Gain1/1
  smooth2/1 -> Saturation11/1
  FB Gain1/1 -> LLoad [F]/1
  dxThigh [m]/1 -> smooth2/1

== system nms_3Dmodel/Body Mechanics Layer/Right Thigh Sensor Sheet ==
  note: Inner Segment Pressure Sheet
  Gain3 : Gain  Gain=k_pressure
  Gain4 : Gain  Gain=1/v_max_pressure
  Inner Thigh Shift Joint : mblibv1/Joints/Prismatic  LConnTagsString=__newl0|SA1|SA2  RConnTagsString=__newr0|SA1  UpdateFromCAD=off  NumSAPorts=3  CutJoint=off  MarkAsCut=off  Primitives=prismatic  PrimitiveProps=P1$WORLD$[1 0 0]$prismatic  DialogClass=JointBlock  P1Axis=[1 0 0]
      settings: SourceProductName=Simscape Multibody  SourceProductBaseCode=MS
  Mux1 : Mux  Inputs=2
  Pressure Sheet Reaction Force : Fcn  Expr=-u(1) * (1+sgn(u(1))*u(2))
  Right Thigh Sensor Sheet IC : mblibv1/Sensors &  Actuators/Joint Initial Condition  UpdateFromCAD=off  LeftPortType=blob  RightPortType=blob  PhysicalDomain=mechanical  DialogClass=InitialConditionBlock  InitialConditions=P1$true$0$m$rad$0$m/s$rad/s#P2$false$0$m$rad$0$m/s$rad/s#P3$false$0$m$rad$0$m/s$rad/s#R1$false$0$m$rad$0$m/s$rad/s#R2$false$0$m$rad$0$m/s$rad/s#R3$false$0$m$rad$0$m/s$rad/s#S$false$0$m$rad$0$m/s$rad/s  P1PIC=0  P1VIC=0  P2PIC=0  P2VIC=0  P3PIC=0  P3VIC=0  R1PIC=0  R1VIC=0  R2PIC=0  R2VIC=0  R3PIC=0  R3VIC=0  SPIC=0  SVIC=0
      settings: SourceProductName=Simscape Multibody  SourceProductBaseCode=MS
  Thigh Actuator : mblibv1/Sensors &  Actuators/Joint Actuator  UpdateFromCAD=off  PhysicalDomain=Mechanical  PortType=blob  ActuationStyle=Force  AngleUnits=deg  ArcVelocityUnits=deg/s  ArcAccelerationUnits=deg/s^2  CoordPositionUnits=m  VelocityUnits=m/s  AccelerationUnits=m/s^2  ForceUnits=N  TorqueUnits=N-m  ActiveIO=on  Width=1  DialogClass=MechanicalActuatorBlock  Primitive=P1  ReferenceFrame=Absolute (INERTIAL)
      settings: SourceProductName=Simscape Multibody  SourceProductBaseCode=MS
  Thigh Sensor : mblibv1/Sensors &  Actuators/Joint Sensor  UpdateFromCAD=off  PhysicalDomain=Mechanical  PortType=blob  Muxed=off  Pose=off  Angle=on  AngleUnits=deg  ArcVelocity=off  ArcVelocityUnits=deg/s  ArcAcceleration=off  ArcAccelerationUnits=deg/s^2  CoordPosition=on  CoordPositionUnits=m  Velocity=on  VelocityUnits=m/s  Acceleration=off  AccelerationUnits=m/s^2  Quaternion=on  QuaternionDT=off  QuaternionDDT=off  QuaternionUnits=off  OutputVector=[ 1 1 ]  ActiveIO=on  Width=2  DialogClass=MechanicalSensorBlock  Primitive=P1  Force=off  ForceUnits=N  Torque=off  TorqueUnits=N-m  ReferenceFrame=Absolute (INERTIAL)  ReactionSensedSide=Base  ReactionReferenceFrame=Absolute (World)  ReactionForce=off  ReactionForceUnits=N  ReactionMoment=off  ReactionMomentUnits=N-m
      settings: SourceProductName=Simscape Multibody  SourceProductBaseCode=MS
  B : PMIOPort  Tag=PMCPort  Port=1  Side=Left
  F : PMIOPort  Tag=PMCPort  Port=2  Side=Right
  dx : Outport
  wires:
  Thigh Sensor/1 -> Gain3/1, dx/1
  Thigh Sensor/2 -> Gain4/1
  Mux1/1 -> Pressure Sheet Reaction Force/1
  Gain3/1 -> Mux1/1
  Gain4/1 -> Mux1/2
  Pressure Sheet Reaction Force/1 -> Thigh Actuator/1
  connections:
  B/RConn1 -- Inner Thigh Shift Joint/LConn1
  F/RConn1 -- Inner Thigh Shift Joint/RConn1
  Thigh Sensor/LConn1 -- Inner Thigh Shift Joint/LConn2
  Inner Thigh Shift Joint/RConn2 -- Thigh Actuator/RConn1
  Inner Thigh Shift Joint/LConn3 -- Right Thigh Sensor Sheet IC/RConn1

== system nms_3Dmodel/Body Mechanics Layer/body pitch//roll//yaw in body frame --- x-axis: forward y-axis: leftward z-axis: parallel to gravity ==
  LHip : Inport
  dLHip : Inport  Port=2
  HAT : Inport  Port=3
  dHAT : Inport  Port=4
  RHip : Inport  Port=5
  dRHip : Inport  Port=6
  " Mean Hip Speed" : Gain  Gain=1/2
  "Dx, Dy" : Selector  InputPortWidth=3  IndexOptions=Index vector (dialog)  Indices=[1 2]  OutputSizes=1
  "Dx, Dz" : Selector  InputPortWidth=3  IndexOptions=Index vector (dialog)  Indices=[1 3]  OutputSizes=1
  "Dx, Dz1" : Selector  InputPortWidth=3  IndexOptions=Index vector (dialog)  Indices=[1 3]  OutputSizes=1
  "Dz, Dy" : Selector  InputPortWidth=3  IndexOptions=Index vector (dialog)  Indices=[3 2]  OutputSizes=1
  Mean Hip Position : Gain  Gain=1/2
  Mux1 : Mux  Inputs=2
  Mux2 : Mux  Inputs=2
  Mux3 : Mux  Inputs=2
  Sum1 : Sum
  Sum2 : Sum
  Sum4 : Sum  Inputs=-+
  Sum5 : Sum  Inputs=+-
  Theta : Fcn  Expr=atan2(u(1),u(2))
  Theta1 : Fcn  Expr=atan2(u(1),u(2))
  "dDx, dDy" : Selector  InputPortWidth=3  IndexOptions=Index vector (dialog)  Indices=[1 2]  OutputSizes=1
  "dDz, dDy" : Selector  InputPortWidth=3  IndexOptions=Index vector (dialog)  Indices=[3 2]  OutputSizes=1
  dTheta : Fcn  Expr=( u(2)*u(3) - u(1)*u(4) ) / D1G_HAT^2
  dTheta1 : Fcn  Expr=( u(2)*u(3) - u(1)*u(4) ) / D1G_HAT^2
  map1 : Subsystem
  map2 : Subsystem
  new_bases : Subsystem
  yaw1 : Fcn  Expr=atan2(-u(1)+u(3),-u(2)+u(4))
  th_pitch : Outport
  dth_pitch : Outport  Port=2
  th_roll : Outport  Port=3
  dth_roll : Outport  Port=4
  yaw : Outport  Port=5
  wires:
  dHAT/1 -> Sum5/1
  "dDx, dDy"/1 -> Mux2/2
  Mux2/1 -> dTheta/1
  Sum1/1 -> Mean Hip Position/1
  Sum2/1 -> " Mean Hip Speed"/1
  HAT/1 -> Sum4/2
  Mean Hip Position/1 -> Sum4/1
  " Mean Hip Speed"/1 -> Sum5/2
  "Dx, Dy"/1 -> Mux2/1, Theta/1
  LHip/1 -> Sum1/1, new_bases/1(L), "Dx, Dz"/1
  RHip/1 -> Sum1/2, new_bases/2(R), "Dx, Dz1"/1
  dLHip/1 -> Sum2/1
  dRHip/1 -> Sum2/2
  Theta/1 -> th_pitch/1
  dTheta/1 -> dth_pitch/1
  Sum4/1 -> map1/1(v)
  map1/1(v_new) -> "Dx, Dy"/1, "Dz, Dy"/1
  new_bases/1(bases) -> map1/2(basis), map2/2(basis)
  Sum5/1 -> map2/1(v)
  map2/1(v_new) -> "dDx, dDy"/1, "dDz, dDy"/1
  "dDz, dDy"/1 -> Mux1/2
  Mux1/1 -> dTheta1/1
  "Dz, Dy"/1 -> Mux1/1, Theta1/1
  Theta1/1 -> th_roll/1
  dTheta1/1 -> dth_roll/1
  "Dx, Dz"/1 -> Mux3/1
  "Dx, Dz1"/1 -> Mux3/2
  Mux3/1 -> yaw1/1
  yaw1/1 -> yaw/1

== system nms_3Dmodel/Body Mechanics Layer/lateral d, v in body frame (left) ==
  body yaw : Inport
  d0 : Inport  Port=2
  dist : Inport  Port=3
  vel : Inport  Port=4
  Mux1 : Mux  Inputs=2
  Mux2 : Mux  Inputs=2
  Mux3 : Mux  Inputs=2
  Sum : Sum  Inputs=-+|
  body frame in transverse plane (xz-plane)1 : Fcn  Expr=u(2)*sin(u(1)) + u(3)*cos(u(1))
  body frame in transverse plane (xz-plane)2 : Fcn  Expr=u(2)*sin(u(1)) + u(3)*cos(u(1))
  "d, v" : Outport
  wires:
  Sum/1 -> Mux1/2
  Mux1/1 -> body frame in transverse plane (xz-plane)1/1
  body yaw/1 -> Mux2/1, Mux1/1
  Mux2/1 -> body frame in transverse plane (xz-plane)2/1
  d0/1 -> Sum/1
  dist/1 -> Sum/2
  body frame in transverse plane (xz-plane)2/1 -> Mux3/2
  vel/1 -> Mux2/2
  body frame in transverse plane (xz-plane)1/1 -> Mux3/1
  Mux3/1 -> "d, v"/1

== system nms_3Dmodel/Body Mechanics Layer/lateral d, v in body frame (right) ==
  body yaw : Inport
  d0 : Inport  Port=2
  dist : Inport  Port=3
  vel : Inport  Port=4
  Mux1 : Mux  Inputs=2
  Mux2 : Mux  Inputs=2
  Mux3 : Mux  Inputs=2
  Sum : Sum  Inputs=-+|
  body frame in transverse plane (xz-plane)1 : Fcn  Expr=u(2)*sin(u(1)) + u(3)*cos(u(1))
  body frame in transverse plane (xz-plane)2 : Fcn  Expr=u(2)*sin(u(1)) + u(3)*cos(u(1))
  "d, v" : Outport
  wires:
  Sum/1 -> Mux1/2
  Mux1/1 -> body frame in transverse plane (xz-plane)1/1
  body yaw/1 -> Mux2/1, Mux1/1
  Mux2/1 -> body frame in transverse plane (xz-plane)2/1
  d0/1 -> Sum/1
  dist/1 -> Sum/2
  body frame in transverse plane (xz-plane)2/1 -> Mux3/2
  vel/1 -> Mux2/2
  body frame in transverse plane (xz-plane)1/1 -> Mux3/1
  Mux3/1 -> "d, v"/1

== system nms_3Dmodel/Body Mechanics Layer/sagittal d, v in body frame (left) ==
  body yaw : Inport
  d0 : Inport  Port=2
  dist : Inport  Port=3
  vel : Inport  Port=4
  Mux1 : Mux  Inputs=2
  Mux2 : Mux  Inputs=2
  Mux3 : Mux  Inputs=2
  Sum : Sum  Inputs=-+|
  body frame in transverse plane (xz-plane)1 : Fcn  Expr=u(2)*cos(u(1)) - u(3)*sin(u(1))
  body frame in transverse plane (xz-plane)2 : Fcn  Expr=u(2)*cos(u(1)) - u(3)*sin(u(1))
  "d, v" : Outport
  tag scope: HAT_Velocity=global
  wires:
  Sum/1 -> Mux1/2
  Mux1/1 -> body frame in transverse plane (xz-plane)1/1
  body yaw/1 -> Mux2/1, Mux1/1
  Mux2/1 -> body frame in transverse plane (xz-plane)2/1
  d0/1 -> Sum/1
  dist/1 -> Sum/2
  vel/1 -> Mux2/2
  body frame in transverse plane (xz-plane)1/1 -> Mux3/1
  Mux3/1 -> "d, v"/1
  body frame in transverse plane (xz-plane)2/1 -> [HAT_Velocity], Mux3/2

== system nms_3Dmodel/Body Mechanics Layer/sagittal d, v in body frame (right) ==
  body yaw : Inport
  d0 : Inport  Port=2
  dist : Inport  Port=3
  vel : Inport  Port=4
  Mux1 : Mux  Inputs=2
  Mux2 : Mux  Inputs=2
  Mux3 : Mux  Inputs=2
  Sum : Sum  Inputs=-+|
  body frame in transverse plane (xz-plane)1 : Fcn  Expr=u(2)*cos(u(1)) - u(3)*sin(u(1))
  body frame in transverse plane (xz-plane)2 : Fcn  Expr=u(2)*cos(u(1)) - u(3)*sin(u(1))
  "d, v" : Outport
  wires:
  Sum/1 -> Mux1/2
  Mux1/1 -> body frame in transverse plane (xz-plane)1/1
  body yaw/1 -> Mux2/1, Mux1/1
  Mux2/1 -> body frame in transverse plane (xz-plane)2/1
  d0/1 -> Sum/1
  dist/1 -> Sum/2
  body frame in transverse plane (xz-plane)2/1 -> Mux3/2
  vel/1 -> Mux2/2
  body frame in transverse plane (xz-plane)1/1 -> Mux3/1
  Mux3/1 -> "d, v"/1

== system nms_3Dmodel/Data Logging/Angles ==
  Mux : Mux  Inputs=8
  Angles : Outport
  wires:
  Mux/1 -> Angles/1
  [Rphi34dphi34] -> Mux/5
  [Lphi12dphi12] -> Mux/4
  [Lphi34dphi34R] -> Mux/2
  [Rphi34dphi34R] -> Mux/6
  [Lphi23dphi23] -> Mux/3
  [Rphi23dphi23] -> Mux/7
  [Lphi34dphi34] -> Mux/1
  [Rphi12dphi12] -> Mux/8

== system nms_3Dmodel/Data Logging/BodyInfo ==
  Angles : Inport
  Postitions : Inport  Port=2
  Loads : Inport  Port=3
  Mux1 : Mux  Inputs=3
  To File8 : ToFile  Filename=Records/BodyInfo
  wires:
  Angles/1 -> Mux1/1
  Mux1/1 -> To File8/1
  Postitions/1 -> Mux1/2
  Loads/1 -> Mux1/3

== system nms_3Dmodel/Data Logging/COMCalculation  ==
  Add4 : Sum  Inputs=9
  Add5 : Sum  Inputs=9
  Constant : Constant  Value=m_HAT/m_Total
  Constant14 : Constant  Value=m_S/m_Total
  Constant16 : Constant  Value=m_F/m_Total
  Constant17 : Constant  Value=m_HAT/m_Total
  Constant18 : Constant  Value=(m_T*(1-ThPos))/m_Total
  Constant19 : Constant  Value=(m_T*(ThPos))/m_Total
  Constant20 : Constant  Value=m_S/m_Total
  Constant21 : Constant  Value=m_F/m_Total
  Constant7 : Constant  Value=(m_T*(1-ThPos))/m_Total
  Constant8 : Constant  Value=(m_T*(ThPos))/m_Total
  Product{,1..17} (18 alike) : Product
  tag scope: dxyzCOM=global, xyzCOM=global
  wires:
  Product4/1 -> Add4/5
  Product6/1 -> Add4/7
  [dxyzLThighHigh] -> Product10/1
  Product11/1 -> Add5/3
  Product8/1 -> Add4/9
  Product14/1 -> Add5/6
  Constant18/1 -> Product10/2, Product11/1
  [xyzLShank] -> Product5/1
  Add5/1 -> [dxyzCOM]
  [dxyzRThighHigh] -> Product11/2
  [dxyzLThighLow] -> Product12/1
  Constant21/1 -> Product16/2, Product17/1
  [xyzHAT] -> Product/1
  [dxyzLFoot] -> Product16/1
  Constant7/1 -> Product2/1, Product1/2
  [xyzLThighHigh] -> Product1/1
  Constant14/1 -> Product5/2, Product6/1
  Add4/1 -> [xyzCOM]
  Product2/1 -> Add4/3
  [dxyzRThighLow] -> Product13/2
  [xyzRFoot] -> Product8/2
  Constant19/1 -> Product12/2, Product13/1
  [xyzLFoot] -> Product7/1
  [dxyzRFoot] -> Product17/2
  Constant16/1 -> Product8/1, Product7/2
  [xyzLThighLow] -> Product3/1
  Product/1 -> Add4/1
  Product17/1 -> Add5/9
  Product13/1 -> Add5/5
  Product9/1 -> Add5/1
  Constant17/1 -> Product9/2
  Product3/1 -> Add4/4
  Product1/1 -> Add4/2
  [xyzRThighLow] -> Product4/2
  [dxyzRShank] -> Product15/2
  Product7/1 -> Add4/8
  Product5/1 -> Add4/6
  Product16/1 -> Add5/8
  Product15/1 -> Add5/7
  Constant8/1 -> Product4/1, Product3/2
  Product10/1 -> Add5/2
  [dxyzHAT] -> Product9/1
  [dxyzLShank] -> Product14/1
  Product12/1 -> Add5/4
  Constant20/1 -> Product15/1, Product14/2
  Constant/1 -> Product/2
  [xyzRShank] -> Product6/2
  [xyzRThighHigh] -> Product2/2

== system nms_3Dmodel/Data Logging/Dist ==
  Mux : Mux  Inputs=8
  Dist : Outport
  wires:
  Mux/1 -> Dist/1
  [xyzHAT_D_sag] -> Mux/1
  [xyzHAT_D_front] -> Mux/2
  [xyzLAnkle_D] -> Mux/3
  [xyzRAnkle_D] -> Mux/4
  [LM34_D] -> Mux/5
  [RM34_D] -> Mux/6
  [LM23_D] -> Mux/7
  [RM23_D] -> Mux/8

== system nms_3Dmodel/Data Logging/Disturbances ==
  Dist : Inport
  To File21 : ToFile  Filename=Records/Disturbance
  wires:
  Dist/1 -> To File21/1

== system nms_3Dmodel/Data Logging/Joint Torques2 ==
  Target : Inport
  To File12 : ToFile  Filename=Records/TargetAngle
  wires:
  Target/1 -> To File12/1

== system nms_3Dmodel/Data Logging/Joint TorquesPassive ==
  LTor : Inport
  RTor : Inport  Port=2
  To File12 : ToFile  Filename=Records/L_Tor_Passive
  To File9 : ToFile  Filename=Records/R_Tor_Passvie
  wires:
  LTor/1 -> To File12/1
  RTor/1 -> To File9/1

== system nms_3Dmodel/Data Logging/Joint TorquesTotal ==
  LTor : Inport
  RTor : Inport  Port=2
  To File12 : ToFile  Filename=Records/L_Tor
  To File9 : ToFile  Filename=Records/R_Tor
  wires:
  RTor/1 -> To File9/1
  LTor/1 -> To File12/1

== system nms_3Dmodel/Data Logging/Knee controller ==
  knee data : Inport
  To File20 : ToFile  Filename=Records/Knee_controller_data  SampleTime=0.001
  wires:
  knee data/1 -> To File20/1

== system nms_3Dmodel/Data Logging/Knee controller1 ==
  knee data : Inport
  To File20 : ToFile  Filename=Records/Knee_buffer  SaveFormat=Timeseries  SampleTime=0.001
  wires:
  knee data/1 -> To File20/1

== system nms_3Dmodel/Data Logging/Loads ==
  Mux : Mux  Inputs=2
  Loads : Outport
  wires:
  Mux/1 -> Loads/1
  [RLLoad] -> Mux/1
  [LLLoad] -> Mux/2

== system nms_3Dmodel/Data Logging/M1 ==
  M11 : Inport
  To File2 : ToFile  Filename=Records/M11
  wires:
  M11/1 -> To File2/1

== system nms_3Dmodel/Data Logging/Muscle Activation1 ==
  L_MA : Inport
  R_MA : Inport  Port=2
  To File1 : ToFile  Filename=Records/R_MA
  To File5 : ToFile  Filename=Records/L_MA
  wires:
  R_MA/1 -> To File1/1
  L_MA/1 -> To File5/1

== system nms_3Dmodel/Data Logging/Muscle Power ==
  L_MA : Inport
  R_MA : Inport  Port=2
  To File1 : ToFile  Filename=Records/R_Power
  To File5 : ToFile  Filename=Records/L_Power
  wires:
  R_MA/1 -> To File1/1
  L_MA/1 -> To File5/1

== system nms_3Dmodel/Data Logging/Positions ==
  Mux : Mux  Inputs=19
  Positions : Outport
  wires:
  Mux/1 -> Positions/1
  [xyzRAnkle] -> Mux/7
  [xyzLKnee] -> Mux/4
  [xyzLHip] -> Mux/5
  [dxyzLHip] -> Mux/6
  [xyzRKnee] -> Mux/8
  [xyzLAnkle] -> Mux/3
  [xyzRHip] -> Mux/9
  [dxyzRHip] -> Mux/10
  [xyzHAT] -> Mux/1
  [dxyzHAT] -> Mux/2
  [xyzTrunk] -> Mux/11
  [xyzLLHeel] -> Mux/12
  [xyzLMHeel] -> Mux/13
  [xyzLLBall] -> Mux/14
  [xyzLMBall] -> Mux/15
  [xyzRLHeel] -> Mux/16
  [xyzRMHeel] -> Mux/17
  [xyzRLBall] -> Mux/18
  [xyzRMBall] -> Mux/19

== system nms_3Dmodel/Data Logging/Sensors ==
  LC : Inport
  RC : Inport  Port=2
  To File19 : ToFile  Filename=Records/L_Clean
  To File20 : ToFile  Filename=Records/R_Clean
  wires:
  LC/1 -> To File19/1
  RC/1 -> To File20/1

== system nms_3Dmodel/Data Logging/Signals NMC Left1 ==
  Mux : Mux
  Target : Outport
  wires:
  [Ralpha_tgt] -> Mux/2
  [RhipR_tgt] -> Mux/4
  [LhipR_tgt] -> Mux/3
  [Lalpha_tgt] -> Mux/1
  Mux/1 -> Target/1

== system nms_3Dmodel/Data Logging/Signals NMC Left2 ==
  Mux : Mux  Inputs=11
  signals : Outport
  wires:
  Mux/1 -> signals/1
  [LStimHFL] -> Mux/1
  [LStimGLU] -> Mux/9
  [LStimVAS] -> Mux/3
  [LStimBFSH] -> Mux/7
  [LStimHAD] -> Mux/11
  [LStimSOL] -> Mux/5
  [LStimHAB] -> Mux/10
  [LStimHAM] -> Mux/8
  [LStimGAS] -> Mux/6
  [LStimTA] -> Mux/4
  [LStimRF] -> Mux/2

== system nms_3Dmodel/Data Logging/Signals NMC Left3 ==
  Mux : Mux
  signals : Outport
  wires:
  Mux/1 -> signals/1
  [LM34] -> Mux/1
  [LM23] -> Mux/3
  [LM12] -> Mux/4
  [LM34R] -> Mux/2

== system nms_3Dmodel/Data Logging/Signals NMC Left4 ==
  Mux : Mux
  signals : Outport
  wires:
  [LHipRStop] -> Mux/2
  [LAnkleStop] -> Mux/4
  [LKneeStop] -> Mux/3
  [LHipStop] -> Mux/1
  Mux/1 -> signals/1

== system nms_3Dmodel/Data Logging/Signals NMC Left6 ==
  Mux : Mux  Inputs=11
  signals : Outport
  wires:
  [REnergyRF] -> Mux/2
  [REnergyTA] -> Mux/4
  [REnergyGAS] -> Mux/6
  [REnergyHAM] -> Mux/8
  [REnergyHAB] -> Mux/10
  [REnergySOL] -> Mux/5
  [REnergyHAD] -> Mux/11
  [REnergyBFSH] -> Mux/7
  [REnergyVAS] -> Mux/3
  [REnergyGLU] -> Mux/9
  [REnergyHFL] -> Mux/1
  Mux/1 -> signals/1

== system nms_3Dmodel/Data Logging/Signals NMC Left7 ==
  Mux : Mux  Inputs=11
  signals : Outport
  wires:
  Mux/1 -> signals/1
  [LEnergyHFL] -> Mux/1
  [LEnergyGLU] -> Mux/9
  [LEnergyVAS] -> Mux/3
  [LEnergyBFSH] -> Mux/7
  [LEnergyHAD] -> Mux/11
  [LEnergySOL] -> Mux/5
  [LEnergyHAB] -> Mux/10
  [LEnergyHAM] -> Mux/8
  [LEnergyGAS] -> Mux/6
  [LEnergyTA] -> Mux/4
  [LEnergyRF] -> Mux/2

== system nms_3Dmodel/Data Logging/Signals NMC Right1 ==
  Mux : Mux
  signals : Outport
  wires:
  [RHipStopR] -> Mux/2
  [RAnkleStop] -> Mux/4
  [RKneeStop] -> Mux/3
  [RHipStop] -> Mux/1
  Mux/1 -> signals/1

== system nms_3Dmodel/Data Logging/Signals NMC Right2 ==
  Mux : Mux  Inputs=11
  signals : Outport
  wires:
  [RStimRF] -> Mux/2
  [RStimTA] -> Mux/4
  [RStimGAS] -> Mux/6
  [RStimHAM] -> Mux/8
  [RStimHAB] -> Mux/10
  [RStimSOL] -> Mux/5
  [RStimHAD] -> Mux/11
  [RStimBFSH] -> Mux/7
  [RStimVAS] -> Mux/3
  [RStimGLU] -> Mux/9
  [RStimHFL] -> Mux/1
  Mux/1 -> signals/1

== system nms_3Dmodel/Data Logging/Signals NMC Right3 ==
  Mux : Mux
  signals : Outport
  wires:
  Mux/1 -> signals/1
  [RM34] -> Mux/1
  [RM23] -> Mux/3
  [RM12] -> Mux/4
  [RM34R] -> Mux/2

== system nms_3Dmodel/Data Logging/SignalsFromNMC_L17 ==
  Mux1 : Mux  Inputs=19
  SigOut : Outport
  wires:
  [LLceHAB] -> Mux1/19
  [LFmHAB] -> Mux1/17
  [LLceHAM] -> Mux1/10
  [LFmHAM] -> Mux1/2
  [LLceTA] -> Mux1/7
  [LFmVAS] -> Mux1/3
  [LLceHFL] -> Mux1/14
  [LFmSOL] -> Mux1/6
  [LFmGLU] -> Mux1/1
  [LLceBFSH] -> Mux1/4
  [LVceRF] -> Mux1/9
  [LLceHAD] -> Mux1/18
  [LVceBFSH] -> Mux1/13
  [LFmGAS] -> Mux1/5
  [LLceGLU] -> Mux1/15
  [LLceRF] -> Mux1/8
  [LVceVAS] -> Mux1/12
  Mux1/1 -> SigOut/1
  [LVceHAM] -> Mux1/11
  [LLceVAS] -> Mux1/16

== system nms_3Dmodel/Data Logging/SignalsFromNMC_L23 ==
  Mux1 : Mux  Inputs=19
  SigOut : Outport
  wires:
  [RLceVAS] -> Mux1/16
  [RVceHAM] -> Mux1/11
  Mux1/1 -> SigOut/1
  [RVceVAS] -> Mux1/12
  [RLceRF] -> Mux1/8
  [RLceGLU] -> Mux1/15
  [RFmGAS] -> Mux1/5
  [RVceBFSH] -> Mux1/13
  [RLceHAD] -> Mux1/18
  [RVceRF] -> Mux1/9
  [RLceBFSH] -> Mux1/4
  [RFmGLU] -> Mux1/1
  [RFmSOL] -> Mux1/6
  [RLceHFL] -> Mux1/14
  [RFmVAS] -> Mux1/3
  [RLceTA] -> Mux1/7
  [RFmHAM] -> Mux1/2
  [RLceHAM] -> Mux1/10
  [RFmHAB] -> Mux1/17
  [RLceHAB] -> Mux1/19

== system nms_3Dmodel/Data Logging/StanceInfo ==
  LStance : Inport
  RStance : Inport  Port=2
  Mux4 : Mux  Inputs=2
  To File4 : ToFile  Filename=Records/StanceSig
  wires:
  Mux4/1 -> To File4/1
  RStance/1 -> Mux4/2
  LStance/1 -> Mux4/1

== system nms_3Dmodel/Data Logging/Subsystem ==
  RotTrunk : Inport
  To File8 : ToFile  Filename=Records/rotTrunk
  wires:
  RotTrunk/1 -> To File8/1

== system nms_3Dmodel/Disturbances/Disturbances ==
  Dist : Inport
  Demux : Demux  Outputs=8
  tag scope: LM23_D=global, LM34_D=global, RM23_D=global, RM34_D=global, xyzHAT_D_front=global, xyzHAT_D_sag=global, xyzLAnkle_D=global, xyzRAnkle_D=global
  wires:
  Demux/1 -> [xyzHAT_D_sag]
  Dist/1 -> Demux/1
  Demux/7 -> [LM23_D]
  Demux/8 -> [RM23_D]
  Demux/4 -> [xyzRAnkle_D]
  Demux/3 -> [xyzLAnkle_D]
  Demux/5 -> [LM34_D]
  Demux/6 -> [RM34_D]
  Demux/2 -> [xyzHAT_D_front]

== system nms_3Dmodel/Disturbances/SampleAndHold ==
  Sample : Inport
  Value : Inport  Port=2
  IC=ic : Memory  LinearizeAsDelay=on
  Switch : Switch  Threshold=0.5  SaturateOnIntegerOverflow=on
  Out : Outport
  wires:
  Sample/1 -> Switch/2
  Switch/1 -> IC=ic/1, Out/1
  IC=ic/1 -> Switch/3
  Value/1 -> Switch/1

== system nms_3Dmodel/Higher Control Layer (Supra Spinal Control)/Double Support ==
  LStance : Inport
  RStance : Inport  Port=2
  Lalpha_tgt : Inport  Port=3
  Lphi34 : Inport  Port=4
  Lphi23 : Inport  Port=5
  LHip_tgt : Inport  Port=6
  Lphi34R : Inport  Port=7
  Ralpha_tgt : Inport  Port=8
  Rphi34 : Inport  Port=9
  Rphi23 : Inport  Port=10
  RHip_tgt : Inport  Port=11
  Rphi34R : Inport  Port=12
  Abs{,1..3} (4 alike) : Abs  ZeroCross=off
  Lalpha' : Fcn  Expr=u(1) - u(2)/2
  Logical Operator1 : Logic  Operator=NOR  AllPortsSameDT=off  OutDataTypeStr=boolean
  Logical Operator2 : Logic  Operator=NOT  AllPortsSameDT=off
  Logical Operator3 : Logic  AllPortsSameDT=off
  Logical Operator4 : Logic  AllPortsSameDT=off
  Logical Operator5 : Logic  AllPortsSameDT=off
  Mux1 : Mux  Inputs=2
  Mux5 : Mux  Inputs=2
  Ralpha' : Fcn  Expr=u(1) - u(2)/2
  Relational Operator : RelationalOperator  Operator=>  ZeroCross=off  RndMeth=Nearest
  Sum{1,3,5,7} (4 alike) : Sum  Inputs=-+|
  Sum2 : Sum  Inputs=++|
  Sum4 : Sum  Inputs=++|
  RonL : Outport
  Flight : Outport  Port=2
  LonR : Outport  Port=3
  wires:
  Lalpha'/1 -> Sum7/2  "Lalpha"
  Mux5/1 -> Lalpha'/1
  Ralpha'/1 -> Sum5/2
  Mux1/1 -> Ralpha'/1
  Sum5/1 -> Abs/1
  Sum7/1 -> Abs1/1
  LStance/1 -> Logical Operator3/1, Logical Operator1/1
  RStance/1 -> Logical Operator3/2, Logical Operator1/2
  Lalpha_tgt/1 -> Sum7/1
  Lphi34/1 -> Mux5/1
  Lphi23/1 -> Mux5/2
  Ralpha_tgt/1 -> Sum5/1
  Rphi34/1 -> Mux1/1
  Rphi23/1 -> Mux1/2
  Logical Operator1/1 -> Flight/1
  LHip_tgt/1 -> Sum1/1
  Lphi34R/1 -> Sum1/2
  Sum1/1 -> Abs2/1
  Abs2/1 -> Sum2/1
  Abs1/1 -> Sum2/2
  Sum2/1 -> Relational Operator/1
  RHip_tgt/1 -> Sum3/1
  Rphi34R/1 -> Sum3/2
  Sum3/1 -> Abs3/1
  Abs/1 -> Sum4/2
  Abs3/1 -> Sum4/1
  Sum4/1 -> Relational Operator/2
  Logical Operator4/1 -> RonL/1
  Logical Operator2/1 -> Logical Operator5/2
  Logical Operator5/1 -> LonR/1
  Relational Operator/1 -> Logical Operator2/1, Logical Operator4/2
  Logical Operator3/1 -> Logical Operator5/1, Logical Operator4/1
